simulink model "LTI_DT_60s_sample"  (R2017a)
settings: Solver=VariableStepAuto  StartTime=0.0  StopTime=18000  RelTol=1e-3  EnableMultiTasking=on
values from neighbouring files (symbols this model uses):
  Aori = eye(no_region)+T*L*(Asys_ori + Bsys*Kv_r)*inv(L)    [Main_Recover.m]
  L = zeros(no_region)    [Asys_ori_Creation.m]
  no_region = numBubbles    (= 50)    [Main_Recover.m]
  root = 39    [Main_Recover.m]
  T = 60    [Main_Recover.m]
settings Model: Creator=yaqiz  LastModifiedBy=Yaqi
settings OptimizationCC: LifeSpan=inf
settings DebuggingCC: SFUnexpectedBacktrackingDiag=warning  SFNoUnconditionalDefaultTransitionDiag=warning  SFExecutionAtInitializationDiag=none
settings GRTTargetCC: TargetLangStandard=C89/C90 (ANSI)  GeneratePreprocessorConditionals=Disable all
settings ConfigComp: CovMetricSettings=dw  CovHtmlReporting=on  CovSaveCumulativeToWorkspaceVar=on  CovSaveSingleToWorkspaceVar=on  CovExternalEMLEnable=off

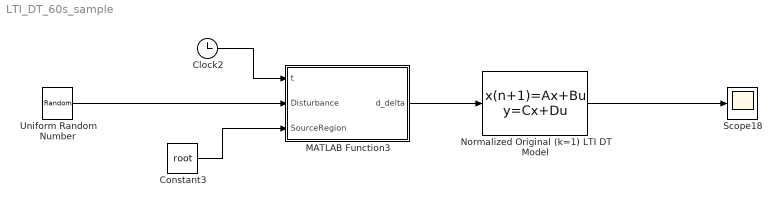
== system LTI_DT_60s_sample ==
  Clock2 : Clock
  Constant3 : Constant  Value=root
  MATLAB Function3 : MATLAB Function  TreatAsAtomicUnit=on
  Normalized Original (k=1) LTI DT Model : DiscreteStateSpace  A=Aori  B=L*T  C=eye(no_region)  D=zeros(no_region)  X0=zeros(no_region,1)  SampleTime=T
  Scope18 : Scope
  Uniform Random Number : UniformRandomNumber  SampleTime=0.1
  wires:
  Normalized Original (k=1) LTI DT Model/1 -> Scope18/1
  Clock2/1 -> MATLAB Function3/1(t)
  Constant3/1 -> MATLAB Function3/3(SourceRegion)
  Uniform Random Number/1 -> MATLAB Function3/2(Disturbance)
  MATLAB Function3/1(d_delta) -> Normalized Original (k=1) LTI DT Model/1

== matlab function LTI_DT_60s_sample/MATLAB Function3 ==
  data: t input; Disturbance input; SourceRegion input; d_delta output size=no_region
function d_delta = fcn(t,Disturbance,SourceRegion)

% coder.varsize('d_delta', [50 1]); %n must never exceed 1024
d_delta = zeros(50,1);

 if t <= 1000000
     d_delta(SourceRegion) = Disturbance;
 end
    
end
